simulink model "tweleve_pulse_rectifier"  (R2019a)
settings: Solver=VariableStepAuto  StartTime=0.0  StopTime=0.02  MaxStep=1e-4  RelTol=1e-3
undefined symbols (not defined in the file): D1, D11, Delta
libraries: powerlib x22
settings Model: Creator=Deepak  LastModifiedBy=Deepak

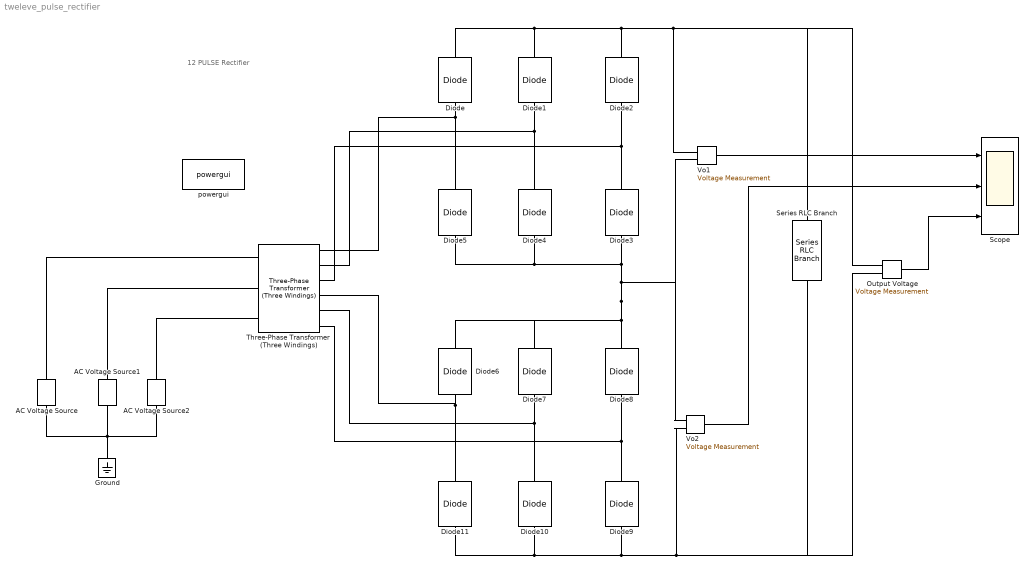
== system tweleve_pulse_rectifier ==
  note: 12 PULSE Rectifier
  AC Voltage Source : powerlib/Electrical Sources/AC Voltage Source  Amplitude=220  Phase=0  Frequency=50  SampleTime=0  Measurements=None  BusType=swing  Pref=10e3  Qref=0  Qmin=-inf  Qmax=+inf
      settings: SourceProductName=Simscape Electrical
  AC Voltage Source1 : powerlib/Electrical Sources/AC Voltage Source  Amplitude=220  Phase=-120  Frequency=50  SampleTime=0  Measurements=None  BusType=swing  Pref=10e3  Qref=0  Qmin=-inf  Qmax=+inf
      settings: SourceProductName=Simscape Electrical
  AC Voltage Source2 : powerlib/Electrical Sources/AC Voltage Source  Amplitude=220  Phase=-240  Frequency=50  SampleTime=0  Measurements=None  BusType=swing  Pref=10e3  Qref=0  Qmin=-inf  Qmax=+inf
      settings: SourceProductName=Simscape Electrical
  Diode{,1..11} (12 alike) : powerlib/Power Electronics/Diode  Ron=0.001  Lon=0  Vf=0  IC=0  UseSnubber=0  Rs=500  Cs=250e-9  Measurements=off
      settings: SourceProductName=Simscape Electrical
  Ground : powerlib/Elements/Ground  LConnTagsString=a
      settings: SourceProductName=Simscape Electrical
  Output Voltage : powerlib/Measurements/Voltage Measurement  PhasorSimulation=off  OutputType=Complex  PSBequivalent=0
      settings: SourceProductName=Simscape Electrical
  Scope : Scope  NumInputPorts=3
  Series RLC Branch : powerlib/Elements/Series RLC Branch  LConnTagsString=__new0  RConnTagsString=__new0  BranchType=R  Resistance=1  Inductance=1e-3  SetiL0=off  InitialCurrent=0  Capacitance=1e-6  Setx0=off  InitialVoltage=0  Measurements=None
      settings: SourceProductName=Simscape Electrical
  Three-Phase Transformer (Three Windings) : powerlib/Elements/Three-Phase Transformer (Three Windings)  Winding1Connection=Delta (D1)  Winding2Connection=Y  Winding3Connection=Delta (D11)  CoreType=Three single-phase transformers  SetSaturation=off  Hysteresis=off  DataFile='hysteresis'  SetInitialFlux=off  Measurements=None  UNITS=pu  NominalPower=[ 250e6 , 50 ]  Winding1=[300 0.02 0]  Winding2=[100 0.02 0]  Winding3=[100 0.02 0]  Rm=500  Lm=500  L0=0.5  Saturation=[ 0,0 ; 0.0024,1.2 ; 1.0,1.52 ]  InitialFluxes=[0.8 -0.8 0.7]  BreakLoop=off  DiscreteSolver=Trapezoidal iterative  DataType=off  TransfoNumber=1
      settings: SourceProductName=Simscape Electrical  SourceProductBaseCode=PS
  Vo1 : powerlib/Measurements/Voltage Measurement  PhasorSimulation=off  OutputType=Complex  PSBequivalent=0
      settings: SourceProductName=Simscape Electrical
  Vo2 : powerlib/Measurements/Voltage Measurement  PhasorSimulation=off  OutputType=Complex  PSBequivalent=0
      settings: SourceProductName=Simscape Electrical
  powergui : powerlib/powergui  Priority=1  SimulationMode=Continuous  SampleTime=50e-6  frequency=60  Iterations=50  frequencyindice=50  Pbase=100e6  ErrMax=1e-4  UnitsV=kV  UnitsW=MW  buscounter=0  FunctionMessages=off  echomessages=off  EnableUseOfTLC=off  CurrentSourceSwitches=off  DisableSnubberDevices=off  DisableRonSwitches=off  DisableVfSwitches=off  DisplayEquations=off  AutomaticDiscreteSolvers=off  SolverType=Tustin/Backward Euler (TBE)  Interpol=off  ExternalGateDelay=off  methode=off  Ts=100  x0status=blocks  SPID=on  SwTol=0  HookPort=off  NonlinearTolerance=0  nMaxIteration=15  ContinueOnMaxIteration=off  RestoreLinks=warning  ResistiveCurrentMeasurement=off  Frange=[0:2:500]  Ylog=off  Xlog=on  ShowGrid=off  save=off  variable=ZData  structure=0  ZoomFFT=off  StartTime=0.0  cycles=1  DisplayStyle=1  fundamental=60  FreqAxis=off  MaxFrequency=1000  frequencyindicesteady=1  RmsSteady=1  display=off
      settings: SourceProductName=Simscape Electrical
  wires:
  Vo1/1 -> Scope/1
  Vo2/1 -> Scope/2
  Output Voltage/1 -> Scope/3
  connections:
  Diode/LConn1 -- Three-Phase Transformer (Three Windings)/RConn1 -- Diode5/RConn1
  Diode1/LConn1 -- Three-Phase Transformer (Three Windings)/RConn2 -- Diode4/RConn1
  Diode2/LConn1 -- Three-Phase Transformer (Three Windings)/RConn3 -- Diode3/RConn1
  Diode/RConn1 -- Diode1/RConn1 -- Vo1/LConn1 -- Series RLC Branch/LConn1 -- Output Voltage/LConn1 -- Diode2/RConn1
  Diode11/LConn1 -- Diode10/LConn1 -- Vo2/LConn2 -- Series RLC Branch/RConn1 -- Output Voltage/LConn2 -- Diode9/LConn1
  Diode5/LConn1 -- Diode4/LConn1 -- Vo2/LConn1 -- Vo1/LConn2 -- Diode8/RConn1 -- Diode7/RConn1 -- Diode6/RConn1 -- Diode3/LConn1
  Diode8/LConn1 -- Three-Phase Transformer (Three Windings)/RConn6 -- Diode9/RConn1
  Diode7/LConn1 -- Three-Phase Transformer (Three Windings)/RConn5 -- Diode10/RConn1
  Diode6/LConn1 -- Diode11/RConn1 -- Three-Phase Transformer (Three Windings)/RConn4
  AC Voltage Source2/RConn1 -- Three-Phase Transformer (Three Windings)/LConn3
  AC Voltage Source1/RConn1 -- Three-Phase Transformer (Three Windings)/LConn2
  AC Voltage Source/RConn1 -- Three-Phase Transformer (Three Windings)/LConn1
  Ground/LConn1 -- AC Voltage Source/LConn1 -- AC Voltage Source2/LConn1 -- AC Voltage Source1/LConn1
